simulink model "PID_na_silnik"  (R2019b)
settings: Solver=VariableStepAuto  StartTime=0.0  StopTime=10.0  RelTol=1e-3
undefined symbols (not defined in the file or in its folder): DiscIntNeverNeededParam
libraries: simulink x1, raspberrypilib x1
settings Model: Creator=damia  LastModifiedBy=damia

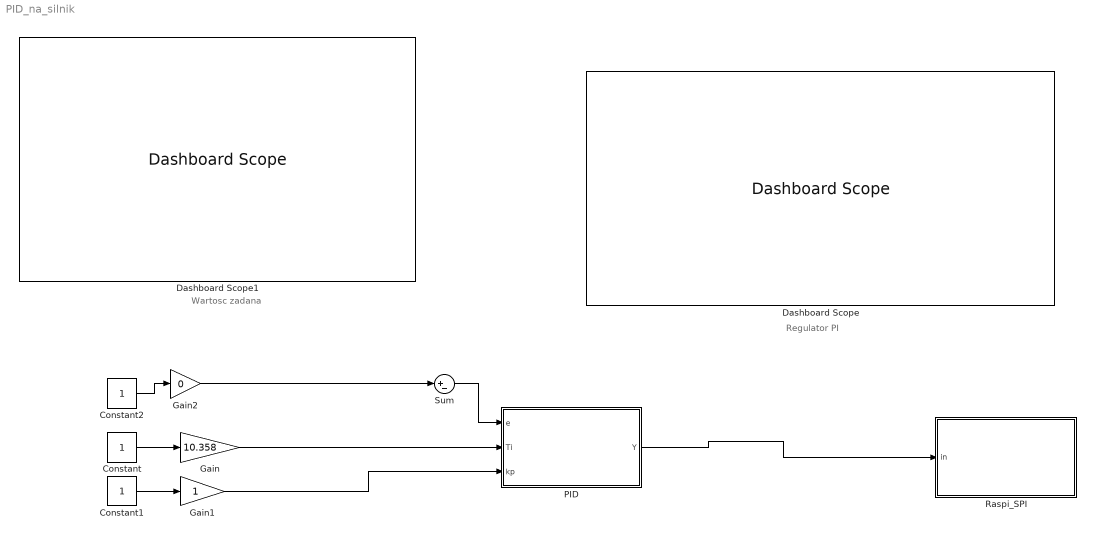
== system PID_na_silnik ==
  note: Wartosc zadana
  note: Regulator PI
  Constant : Constant
  Constant1 : Constant
  Constant2 : Constant
  Dashboard Scope : DashboardScope
  Dashboard Scope1 : DashboardScope
  Gain : Gain  Gain=10.358
  Gain1 : Gain
  Gain2 : Gain  Gain=0
  PID : Subsystem
  Raspi_SPI : Subsystem
  Sum : Sum  Inputs=|+-
  wires:
  Constant1/1 -> Gain1/1
  Sum/1 -> PID/1("e ")
  Constant/1 -> Gain/1
  Gain1/1 -> PID/3(kp)
  Gain/1 -> PID/2(Ti)
  Gain2/1 -> Sum/1
  Constant2/1 -> Gain2/1
  PID/1(Y) -> Raspi_SPI/1("in ")

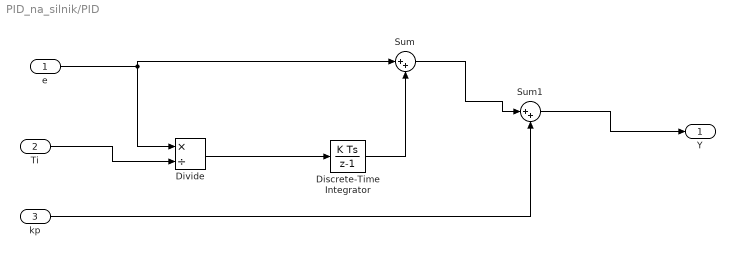
== system PID_na_silnik/PID ==
  "e " : Inport
  Ti : Inport  Port=2
  kp : Inport  Port=3
  Discrete-Time Integrator : DiscreteIntegrator  SampleTime=0.01  ICPrevOutput=DiscIntNeverNeededParam  ICPrevScaledInput=DiscIntNeverNeededParam
  Divide : Product  Inputs=*/
  Sum : Sum  Inputs=|++
  Sum1 : Sum  Inputs=|++
  Y : Outport
  wires:
  "e "/1 -> Sum/1, Divide/1
  Ti/1 -> Divide/2
  Divide/1 -> Discrete-Time Integrator/1
  Discrete-Time Integrator/1 -> Sum/2
  Sum/1 -> Sum1/1
  Sum1/1 -> Y/1
  kp/1 -> Sum1/2

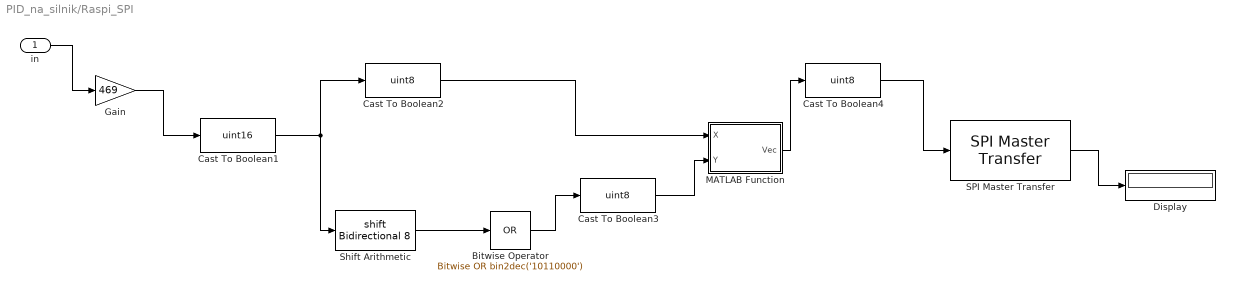
== system PID_na_silnik/Raspi_SPI ==
  "in " : Inport
  Bitwise Operator : simulink/Logic and Bit Operations/Bitwise Operator  logicop=OR  UseBitMask=on  BitMask=bin2dec('10110000')  BitMaskRealWorld=Real World Value
  Cast To Boolean1 : DataTypeConversion  OutDataTypeStr=uint16
  Cast To Boolean2 : DataTypeConversion  OutDataTypeStr=uint8
  Cast To Boolean3 : DataTypeConversion  OutDataTypeStr=uint8
  Cast To Boolean4 : DataTypeConversion  OutDataTypeStr=uint8
  Display : Display
  Gain : Gain  Gain=469
  MATLAB Function : MATLAB Function  TreatAsAtomicUnit=on
  SPI Master Transfer : raspberrypilib/SPI Master Transfer  Priority=1  BoardProperty=Pi 3 Model B  SPIModule=uint32(0)  Mode=Master  BusSpeed=1000000  Pin=SPI0_CE0  FirstBitToTransfer=Most significant bit (MSB)  ClockMode=0  BlockFunction=Transfer  RegisterAddress=0  OutputDataType=int8  OutputDataLength=1
      settings: SourceProductName=Simulink Support Package for Raspberry Pi Hardware  SourceProductBaseCode=RASPPI
  Shift Arithmetic : ArithShift  BitShiftNumber=8
  wires:
  SPI Master Transfer/1 -> Display/1
  MATLAB Function/1(Vec) -> Cast To Boolean4/1
  Cast To Boolean2/1 -> MATLAB Function/1(X)
  Shift Arithmetic/1 -> Bitwise Operator/1
  Bitwise Operator/1 -> Cast To Boolean3/1
  Cast To Boolean4/1 -> SPI Master Transfer/1
  Cast To Boolean3/1 -> MATLAB Function/2(Y)
  Cast To Boolean1/1 -> Cast To Boolean2/1, Shift Arithmetic/1
  Gain/1 -> Cast To Boolean1/1
  "in "/1 -> Gain/1

== matlab function PID_na_silnik/Raspi_SPI/MATLAB Function ==
  data: X input; Vec output; Y input
function Vec = Vector(X, Y)

% myPI = raspi();
Vec = [Y X];
% mySPI = spidev(myPI,'CE0');
% out = writeRead(mySPI,[Vec]);
